simulink model "standalone_propulsion_model"  (R2017b)
settings: Solver=ode4  StartTime=0.0  StopTime=end_time  FixedStep=simm.dt  RelTol=1e-3
values from neighbouring files (symbols this model uses):
  simm = evalin('base','simm')    [model_proplsn_perf_hifi.m]
undefined symbols (not defined in the file or in its folder): proplsn
libraries: proplsn_lib x1
settings Model: Creator=Kevin  LastModifiedBy=Kevin
settings DataIOCC: ExternalInput=[throttle, airspeed_m_s, density_kg_m3]  LoadExternalInput=on  SignalLogging=off  DSMLogging=off
settings CodeAppCC: StateflowObjectComments=on

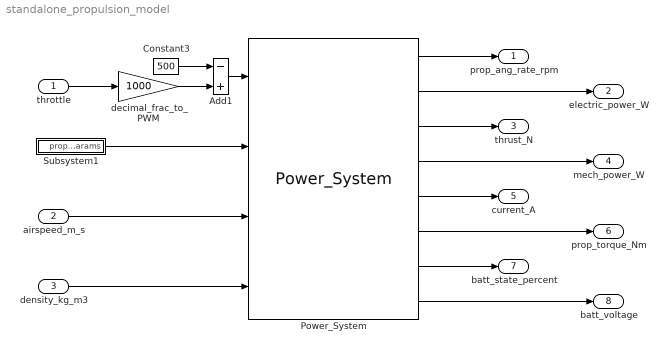
== system standalone_propulsion_model ==
  throttle : Inport  OutMin=0  OutMax=1
  airspeed_m_s : Inport  Port=2
  density_kg_m3 : Inport  Port=3
  Add1 : Sum  Inputs=-+
  Constant3 : Constant  Value=500
  Power_System : proplsn_lib/Power_System
  Subsystem1 : Subsystem
  decimal_frac_to_PWM : Gain  Gain=1000
  prop_ang_rate_rpm : Outport  SampleTime=simm.output_dt
  electric_power_W : Outport  Port=2  SampleTime=simm.output_dt
  thrust_N : Outport  Port=3  SampleTime=simm.output_dt
  mech_power_W : Outport  Port=4  SampleTime=simm.output_dt
  current_A : Outport  Port=5  SampleTime=simm.output_dt
  prop_torque_Nm : Outport  Port=6  SampleTime=simm.output_dt
  batt_state_percent : Outport  Port=7  SampleTime=simm.output_dt
  batt_voltage : Outport  Port=8
  wires:
  throttle/1 -> decimal_frac_to_PWM/1
  Power_System/1 -> prop_ang_rate_rpm/1
  Subsystem1/1(prop_params) -> Power_System/2
  airspeed_m_s/1 -> Power_System/3
  density_kg_m3/1 -> Power_System/4
  Power_System/2 -> electric_power_W/1
  Power_System/3 -> thrust_N/1
  Power_System/4 -> mech_power_W/1
  Power_System/5 -> current_A/1
  Power_System/6 -> prop_torque_Nm/1
  Power_System/7 -> batt_state_percent/1
  Constant3/1 -> Add1/1
  decimal_frac_to_PWM/1 -> Add1/2
  Add1/1 -> Power_System/1
  Power_System/8 -> batt_voltage/1

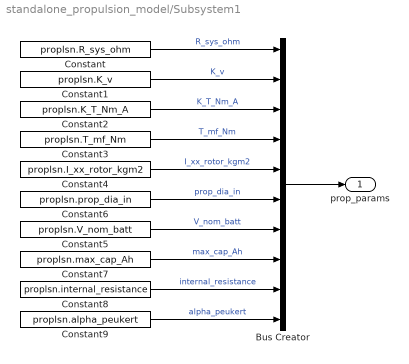
== system standalone_propulsion_model/Subsystem1 ==
  Bus Creator : BusCreator  Inputs=10
  Constant : Constant  Value=proplsn.R_sys_ohm
  Constant1 : Constant  Value=proplsn.K_v
  Constant2 : Constant  Value=proplsn.K_T_Nm_A
  Constant3 : Constant  Value=proplsn.T_mf_Nm
  Constant4 : Constant  Value=proplsn.I_xx_rotor_kgm2
  Constant5 : Constant  Value=proplsn.V_nom_batt
  Constant6 : Constant  Value=proplsn.prop_dia_in
  Constant7 : Constant  Value=proplsn.max_cap_Ah
  Constant8 : Constant  Value=proplsn.internal_resistance
  Constant9 : Constant  Value=proplsn.alpha_peukert
  prop_params : Outport
  wires:
  Bus Creator/1 -> prop_params/1
  Constant/1 -> Bus Creator/1  "R_sys_ohm"
  Constant1/1 -> Bus Creator/2  "K_v"
  Constant2/1 -> Bus Creator/3  "K_T_Nm_A"
  Constant3/1 -> Bus Creator/4  "T_mf_Nm"
  Constant4/1 -> Bus Creator/5  "I_xx_rotor_kgm2"
  Constant5/1 -> Bus Creator/7  "V_nom_batt"
  Constant6/1 -> Bus Creator/6  "prop_dia_in"
  Constant7/1 -> Bus Creator/8  "max_cap_Ah"
  Constant8/1 -> Bus Creator/9  "internal_resistance"
  Constant9/1 -> Bus Creator/10  "alpha_peukert"
